simulink model "pr631_phase_detector"  (R2018b)
settings: Solver=VariableStepAuto  StartTime=0.0  StopTime=1e-3  RelTol=1e-3  EnableMultiTasking=on
PreLoadFcn:
  | fs=200e6;
settings Model: Creator=GRIHA  LastModifiedBy=Григорий Фокин
settings DataIOCC: LimitDataPoints=on
settings OptimizationCC: LifeSpan=inf
settings DebuggingCC: AllowSymbolicDim=off  SFUnexpectedBacktrackingDiag=warning  SFNoUnconditionalDefaultTransitionDiag=warning  SFExecutionAtInitializationDiag=none
settings ModelReferenceCC: PropagateSignalLabelsOutOfModel=off
settings SFSimCC: SimUseLocalCustomCode=off
settings RTWCC: RTWUseLocalCustomCode=off
settings CodeAppCC: StateflowObjectComments=on
settings GRTTargetCC: TargetLangStandard=C89/C90 (ANSI)
settings ConfigComp: CovMetricSettings=dw  CovHtmlReporting=on  CovSaveCumulativeToWorkspaceVar=on  CovSaveSingleToWorkspaceVar=on  CovExternalEMLEnable=off

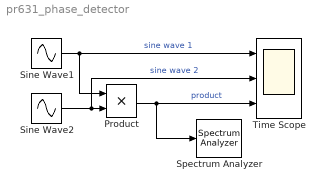
== system pr631_phase_detector ==
  Product : Product
  Sine Wave1 : Sin  Frequency=2*pi*(fs/20)  SampleTime=1/fs
  Sine Wave2 : Sin  Frequency=2*pi*(fs*1.00/20)  Phase=pi/3  SampleTime=1/fs
  Spectrum Analyzer : SpectrumAnalyzer
  Time Scope : Scope  NumInputPorts=3
  wires:
  Sine Wave1/1 -> Product/1, Time Scope/1  "sine wave 1"
  Sine Wave2/1 -> Time Scope/2, Product/2  "sine wave 2"
  Product/1 -> Time Scope/3, Spectrum Analyzer/1  "product"
